simulink model "Kalman_Project"  (R2023a)
settings: Solver=ode45  StartTime=0  StopTime=25  FixedStep=0.002  RelTol=1e-3  AbsTol=1e-6
undefined symbols (not defined in the file or in its folder): J, Reff
libraries: Solver_SF x1, cstblocks x1
settings Model: PacingRate=10  ExtModeTrigMode=oneshot  Creator=ywata  LastModifiedBy=cheho
settings SolverCC: AutoScaleAbsTol=off  AlgebraicLoopSolver=TrustRegion
settings DataIOCC: SaveFormat=Array  SignalLoggingSaveFormat=ModelDataLogs  ReturnWorkspaceOutputs=off  SignalLoggingName=sigsOut
settings OptimizationCC: BlockReduction=off  BooleanDataType=off  ExpressionDepthLimit=2147483647  LifeSpan=inf
settings DebuggingCC: SaveWithParameterizedLinksMsg=none  UnderspecifiedInitializationDetection=Classic  MergeDetectMultiDrivingBlocksExec=none  SignalResolutionControl=TryResolveAllWithWarning  MultiTaskDSMMsg=warning  MultiTaskCondExecSysMsg=none  FcnCallInpInsideContextMsg=warning  UnconnectedInputMsg=warning  UnconnectedOutputMsg=warning  UnconnectedLineMsg=warning  StateNameClashWarn=warning  SFUnexpectedBacktrackingDiag=warning  SFNoUnconditionalDefaultTransitionDiag=warning  SFExecutionAtInitializationDiag=none  ArithmeticOperatorsInVariantConditions=warning
settings HardwareCC: ProdBitPerPointer=32  ProdBitPerSizeT=32  ProdBitPerPtrDiffT=32  ProdLargestAtomicFloat=None  ProdIntDivRoundTo=Undefined  ProdEndianess=Unspecified  ProdWordSize=32  ProdHWDeviceType=32-bit Generic  TargetUnknown=on
settings ModelReferenceCC: PropagateSignalLabelsOutOfModel=off
settings SFSimCC: SimUseLocalCustomCode=off  CustomCodeUndefinedFunction=UseInterfaceOnly
settings RTWCC: TemplateMakefile=grt_vc.tmf  RTWUseLocalCustomCode=off
settings CodeAppCC: StateflowObjectComments=on
settings GRTTargetCC: TargetFcnLib=ansi_tfl_tmw.mat  TargetLangStandard=C89/C90 (ANSI)  CombineOutputUpdateFcns=off  GRTInterface=on
settings ConfigComp: CovMetricSettings=dw  CovSaveCumulativeToWorkspaceVar=on  CovSaveSingleToWorkspaceVar=on  CovExternalEMLEnable=off

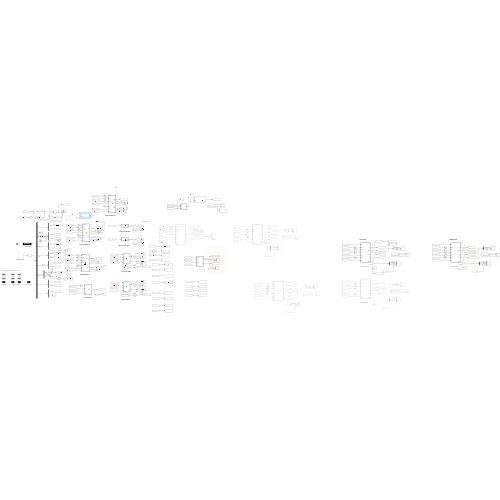
[thumbnail: Simulink's stored preview of the top-level diagram]
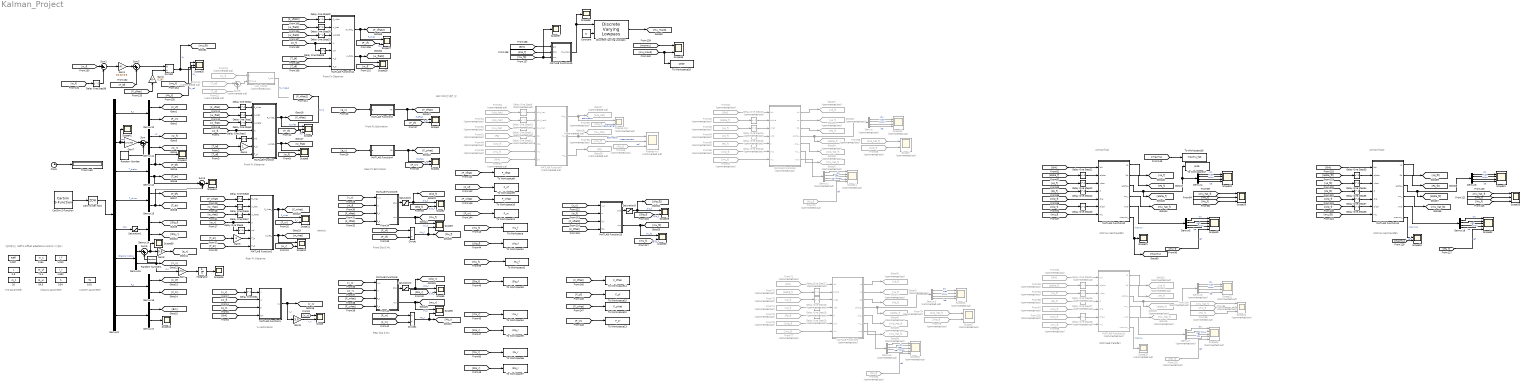
== system Kalman_Project ==
  note: Almost final
  note: IMM(no road transfer)
  note: !실차에서는 Reff와 Offset adaptation control이 필요.!
  note: EKF IMM만 짜면 됨.
  note: Vx estimation
  note: velocity
  note: chassis parameter
  note: tire parameter
  note: system parameter
  note: Front Fx Observer
  note: Rear Fx Observer
  note: Front Fz Estimation
  note: Rear Fz Estimation
  note: Front Slip & Mu
  note: Rear Slip & Mu
  note: IMM(road transfer)
  note: Front Fx Observer
  note: Almost final2
  note: IMM(no road transfer)
  0.01 : DataStoreMemory  DataStoreName=Ts  WriteAfterWriteMsg=warning  InitialValue=0.01  ShowAdditionalParam=off  OutDataTypeStr=double
  0.287 : DataStoreMemory  DataStoreName=Reff  WriteAfterWriteMsg=warning  InitialValue=0.287  ShowAdditionalParam=off  OutDataTypeStr=double
  0.54 : DataStoreMemory  DataStoreName=h  WriteAfterWriteMsg=warning  InitialValue=0.54  ShowAdditionalParam=off  OutDataTypeStr=double
  0.8 : DataStoreMemory  DataStoreName=J  WriteAfterWriteMsg=warning  InitialValue=0.8  ShowAdditionalParam=off  OutDataTypeStr=double
  1.040 : DataStoreMemory  DataStoreName=l_f  WriteAfterWriteMsg=warning  InitialValue=1.040  ShowAdditionalParam=off  OutDataTypeStr=double
  1.560 : DataStoreMemory  DataStoreName=l_r  WriteAfterWriteMsg=warning  InitialValue=1.560  ShowAdditionalParam=off  OutDataTypeStr=double
  1134 : DataStoreMemory  DataStoreName=m_s  WriteAfterWriteMsg=warning  InitialValue=1134  ShowAdditionalParam=off  OutDataTypeStr=double
  16 : DataStoreMemory  DataStoreName=m_t  WriteAfterWriteMsg=warning  InitialValue=16  ShowAdditionalParam=off  OutDataTypeStr=double
  54.5 : DataStoreMemory  DataStoreName=m_ur  WriteAfterWriteMsg=warning  InitialValue=54.5  ShowAdditionalParam=off  OutDataTypeStr=double
  71.4 : DataStoreMemory  DataStoreName=m_uf  WriteAfterWriteMsg=warning  InitialValue=71.4  ShowAdditionalParam=off  OutDataTypeStr=double
  CarSim S-Function : Solver_SF/CarSim S-Function  Priority=1  SIMFILE=simfile.sim  Run_RTs=off  vs_state_ind=Run  StopMode_ind=Vehicle Model
  Clock : Clock
  Constant : Constant  Value=5
  Delay One Step{,1..2,4..6,8,29..30,32,38} (11 alike) : Delay  DelayLength=1
  Delay One Step10 : Delay  Commented=on
  Delay One Step11 : Delay  Commented=on  DelayLength=1
  Delay One Step12 : Delay  Commented=on  DelayLength=1  InitialCondition=[0 0;0 0]
  Delay One Step13 : Delay  Commented=on  DelayLength=1  InitialCondition=[0.25 0.25 0.25 0.25]'
  Delay One Step{14..15,18..19} (4 alike) : Delay  Commented=on  DelayLength=1  InitialCondition=[0 0 0 0;0 0 0 0]
  Delay One Step16 : Delay  Commented=on  DelayLength=1  InitialCondition=[0 0 0 0 0 0 0 0;0 0 0 0 0 0 0 0]
  Delay One Step17 : Delay  Commented=on  DelayLength=1  InitialCondition=[0.25 0.25 0.25 0.25]'
  Delay One Step20 : Delay  Commented=on  DelayLength=1  InitialCondition=[0 0 0 0 0 0 0 0;0 0 0 0 0 0 0 0]
  Delay One Step21 : Delay  DelayLength=1  InitialCondition=[0.25 0.25 0.25 0.25]'
  Delay One Step{22,24..25,34..35,37} (6 alike) : Delay  DelayLength=1  InitialCondition=0
  Delay One Step23 : Delay  Commented=on  DelayLength=1  InitialCondition=[0.25 0.25 0.25 0.25]'
  Delay One Step26 : Delay  Commented=on  DelayLength=1  InitialCondition=0
  Delay One Step27 : Delay  Commented=on  DelayLength=1  InitialCondition=0
  Delay One Step28 : Delay  Commented=on  DelayLength=1  InitialCondition=0
  Delay One Step3 : Delay
  Delay One Step31 : Delay
  Delay One Step33 : Delay  DelayLength=1  InitialCondition=[0.25 0.25 0.25 0.25]'
  Delay One Step36 : Delay  InitialCondition=0
  Delay One Step7 : Delay
  Delay One Step9 : Delay  Commented=on  DelayLength=1
  Demux{,1..3,6..7} (6 alike) : Demux  Commented=on
  Demux{10..17} (8 alike) : Demux  Outputs=[1 1]
      settings: DisplayOption=none
  Demux{4..5,8,18} (4 alike) : Demux
  Demux9 : Demux  Outputs=[2 2 2 2 2 2 2 2]
      settings: DisplayOption=none
  Discrete Varying Lowpass : cstblocks/Linear Parameter Varying/Discrete Varying Lowpass  N=1  w0=0  Ts=0.01
  Divide : Product  Inputs=*/
  Divide1 : Product  Inputs=*/
  Divide2 : Product  Inputs=*/
  From100 : From  Commented=on  GotoTag=mu_hat_f
  From{58,70,80,99,101} (5 alike) : From  Commented=on  GotoTag=Mu_f
  From{49,55,66,68,76,78,97,102} (8 alike) : From  Commented=on  GotoTag=slip_f
  From13 : From  Commented=on  GotoTag=w_f
  From14 : From  Commented=on  GotoTag=T_bf
  From15 : From  Commented=on  GotoTag=T_df
  From{50,56,67,77,95,98} (6 alike) : From  Commented=on  GotoTag=mu_f
  From51 : From  Commented=on  GotoTag=Pp
  From52 : From  Commented=on  GotoTag=mu_hat
  From53 : From  Commented=on  GotoTag=slip_hat
  From54 : From  Commented=on  GotoTag=slip_hat
  From{57,61,71,92} (4 alike) : From  Commented=on  GotoTag=Brk
  From62 : From  Commented=on  GotoTag=alpha_f
  From63 : From  Commented=on  GotoTag=xp_f
  From64 : From  Commented=on  GotoTag=xd_f
  From65 : From  Commented=on  GotoTag=Pp_f
  From69 : From  Commented=on  GotoTag=slip_hat_f
  From72 : From  Commented=on  GotoTag=alpha_f
  From73 : From  Commented=on  GotoTag=xp_f
  From74 : From  Commented=on  GotoTag=xd_f
  From75 : From  Commented=on  GotoTag=Pp_f
  From79 : From  Commented=on  GotoTag=slip_hat_f
  From93 : From  Commented=on  GotoTag=alpha_f
  From94 : From  Commented=on  GotoTag=xp_f
  From96 : From  Commented=on  GotoTag=Pp_f
  Gain : Gain  Gain=1/3.6
  Gain1 : Gain  Gain=1/0.01*0.8
  Gain2 : Gain  Gain=0.287
  Gain3 : Gain
  Gain4 : Gain
  Gain7 : Gain  Gain=2*pi/60
  Gain8 : Gain  Gain=9.8
  Gain9 : Gain  Gain=3.6
  Goto27 : Goto  Commented=on  GotoTag=slip_hat
  Goto28 : Goto  Commented=on  GotoTag=mu_hat
  Goto29 : Goto  Commented=on  GotoTag=Pp
  Goto32 : Goto  Commented=on  GotoTag=mu_hat_f
  Goto33 : Goto  Commented=on  GotoTag=slip_hat_f
  Goto34 : Goto  Commented=on  GotoTag=alpha_f
  Goto35 : Goto  Commented=on  GotoTag=Pp_f
  Goto36 : Goto  Commented=on  GotoTag=xp_f
  Goto37 : Goto  Commented=on  GotoTag=xd_f
  Goto38 : Goto  Commented=on  GotoTag=mu_hat_f
  Goto39 : Goto  Commented=on  GotoTag=slip_hat_f
  Goto40 : Goto  Commented=on  GotoTag=alpha_f
  Goto41 : Goto  Commented=on  GotoTag=Pp_f
  Goto42 : Goto  Commented=on  GotoTag=xp_f
  Goto43 : Goto  Commented=on  GotoTag=xd_f
  Goto45 : Goto  Commented=on  GotoTag=mu_hat_f
  Goto49 : Goto  Commented=on  GotoTag=alpha_f
  Goto50 : Goto  Commented=on  GotoTag=Pp_f
  Goto51 : Goto  Commented=on  GotoTag=xp_f
  Integrator : Integrator
  MATLAB Function : MATLAB Function  TreatAsAtomicUnit=on
  MATLAB Function1 : MATLAB Function  TreatAsAtomicUnit=on
  MATLAB Function10 : MATLAB Function  TreatAsAtomicUnit=on
  MATLAB Function11 : MATLAB Function  Commented=on  TreatAsAtomicUnit=on
  MATLAB Function12 : MATLAB Function  TreatAsAtomicUnit=on
  MATLAB Function13 : MATLAB Function  TreatAsAtomicUnit=on
  MATLAB Function14 : MATLAB Function  TreatAsAtomicUnit=on
  MATLAB Function15 : MATLAB Function  TreatAsAtomicUnit=on
  MATLAB Function2 : MATLAB Function  TreatAsAtomicUnit=on
  MATLAB Function3 : MATLAB Function  TreatAsAtomicUnit=on
  MATLAB Function4 : MATLAB Function  TreatAsAtomicUnit=on
  MATLAB Function5 : MATLAB Function  TreatAsAtomicUnit=on
  MATLAB Function6 : MATLAB Function  TreatAsAtomicUnit=on
  MATLAB Function7 : MATLAB Function  Commented=on  TreatAsAtomicUnit=on
  MATLAB Function8 : MATLAB Function  Commented=on  TreatAsAtomicUnit=on
  MATLAB Function9 : MATLAB Function  Commented=on  TreatAsAtomicUnit=on
  Random Number : RandomNumber  Variance=0.01^2  SampleTime=0.01
  Random Number1 : RandomNumber  Variance=2.25e-8  SampleTime=0.01
  Saturation{,1..3} (4 alike) : Saturate  UpperLimit=1  LowerLimit=-1
  Scope{,1..6,9,11..12,28..30,34,36} (15 alike) : Scope  NumInputPorts=2
  Scope{10,21,26,37..42} (9 alike) : Scope
  Scope13 : Scope  Commented=on  NumInputPorts=4
  Scope14 : Scope  Commented=on  NumInputPorts=5
  Scope15 : Scope  Commented=on  NumInputPorts=4
  Scope16 : Scope  Commented=on  NumInputPorts=5
  Scope17 : Scope  Commented=on  NumInputPorts=2
  Scope18 : Scope  NumInputPorts=4
  Scope19 : Scope  NumInputPorts=5
  Scope{8,20,27,33,35} (5 alike) : Scope  NumInputPorts=3
  Scope22 : Scope  Commented=on  NumInputPorts=4
  Scope23 : Scope  Commented=on  NumInputPorts=5
  Scope24 : Scope  Commented=on  NumInputPorts=3
  Scope25 : Scope  Commented=on
  Scope31 : Scope  NumInputPorts=4
  Scope32 : Scope  NumInputPorts=5
  Scope7 : Scope  Commented=on  NumInputPorts=2
  Sum{,2..3,5} (4 alike) : Sum  Inputs=|++
  Sum1 : Sum  Inputs=|+-
  Sum8 : Sum  Commented=on  Inputs=|++
  Time (sec) : Display
      settings: Format=bank  Decimation=100
  To Workspace : ToWorkspace  VariableName=mu_f  SaveFormat=Timeseries  SampleTime=-1
  To Workspace1 : ToWorkspace  VariableName=slip_f  SaveFormat=Timeseries  SampleTime=-1
  To Workspace10 : ToWorkspace  VariableName=F_xrhat  SaveFormat=Timeseries  SampleTime=-1
  To Workspace11 : ToWorkspace  VariableName=F_xr  SaveFormat=Timeseries  SampleTime=-1
  To Workspace12 : ToWorkspace  VariableName=F_zrhat  SaveFormat=Timeseries  SampleTime=-1
  To Workspace13 : ToWorkspace  VariableName=F_zr  SaveFormat=Timeseries  SampleTime=-1
  To Workspace14 : ToWorkspace  VariableName=F_zfhat  SaveFormat=Timeseries  SampleTime=-1
  To Workspace15 : ToWorkspace  VariableName=F_zf  SaveFormat=Timeseries  SampleTime=-1
  To Workspace16 : ToWorkspace  VariableName=maxmu_hat  SaveFormat=Timeseries  SampleTime=-1
  To Workspace17 : ToWorkspace  VariableName=prob  SaveFormat=Timeseries  SampleTime=-1
  To Workspace18 : ToWorkspace  VariableName=other  SaveFormat=Timeseries  SampleTime=-1
  To Workspace2 : ToWorkspace  VariableName=Mu_f  SaveFormat=Timeseries  SampleTime=-1
  To Workspace3 : ToWorkspace  VariableName=Slip_f  SaveFormat=Timeseries  SampleTime=-1
  To Workspace4 : ToWorkspace  VariableName=mu_r  SaveFormat=Timeseries  SampleTime=-1
  To Workspace5 : ToWorkspace  VariableName=slip_r  SaveFormat=Timeseries  SampleTime=-1
  To Workspace6 : ToWorkspace  VariableName=Mu_r  SaveFormat=Timeseries  SampleTime=-1
  To Workspace7 : ToWorkspace  VariableName=Slip_r  SaveFormat=Timeseries  SampleTime=-1
  To Workspace8 : ToWorkspace  VariableName=F_xfhat  SaveFormat=Timeseries  SampleTime=-1
  To Workspace9 : ToWorkspace  VariableName=F_xf  SaveFormat=Timeseries  SampleTime=-1
  UIO_front2 : Subsystem  Commented=on
  Zero-Order Hold : ZeroOrderHold  SampleTime=0.01
  filtered mu : Scope  Commented=on  NumInputPorts=3
  filtered slip : Scope  Commented=on  NumInputPorts=2
  wires:
  Clock/1 -> Time (sec)/1
  CarSim S-Function/1 -> Zero-Order Hold/1
  Zero-Order Hold/1 -> Demux9/1
  Demux9/1 -> Demux10/1  "F_x"
  Demux10/1 -> [F_xf]
  Demux10/2 -> [F_xr]
  Demux11/2 -> [w_r]
  Demux11/1 -> [w_f]  "wk"
  Demux9/2 -> Scope42/1, Gain7/1  "rpm"
  Gain7/1 -> Sum/1
  Demux12/1 -> Scope40/1, [T_bf]
  Demux12/2 -> Sum3/1, [T_br]
  Demux9/3 -> Demux12/1  "T_brake"
  Demux13/2 -> Sum3/2, [T_dr]
  Demux13/1 -> [T_df]
  Demux9/4 -> Demux13/1  "T_drive"
  Demux14/2 -> [Slip_r]
  Demux14/1 -> [Slip_f]
  Demux9/5 -> Saturation1/1  "slip"
  Demux15/2 -> Gain/1, [V_x]  "V_x"
  Demux15/1 -> Sum5/1
  Demux9/6 -> Demux15/1  "Chassis motion"
  Demux16/2 -> [F_zr]
  Demux16/1 -> [F_zf]
  Demux9/7 -> Demux16/1  "F_z"
  Sum5/1 -> Scope39/1, Gain8/1
  Gain8/1 -> [a_x]
  [w_f] -> MATLAB Function1/2(w)
  [a_x] -> MATLAB Function1/3(a)
  [Brk] -> MATLAB Function1/4(brk)
  Demux9/8 -> Demux17/1
  MATLAB Function1/1(Vx) -> Gain9/1, [v_x]  "v_x"
  [v_x] -> Delay One Step/1
  Delay One Step/1 -> MATLAB Function1/1(v)
  Gain9/1 -> Scope/2  "v_x"
  [V_x] -> Scope/1
  Delay One Step1/1 -> MATLAB Function/5(wd)
  [w_f] -> MATLAB Function/4(w), Delay One Step1/1
  MATLAB Function/2(w_hat_) -> Scope9/1, [w_fhat]
  Delay One Step3/1 -> MATLAB Function/3(w_hatd)
  MATLAB Function/1(F_xhat_) -> Scope8/1, [F_xfhat]  "F_xhat"
  [F_xfhat] -> Delay One Step4/1
  [F_xf] -> Scope8/3  "F_x"
  [w_fhat] -> Delay One Step2/1
  Delay One Step2/1 -> MATLAB Function/2(w_hat)
  Delay One Step4/1 -> MATLAB Function/1(F_xhat)
  Demux17/1 -> [Brk]
  Demux17/2 -> Scope10/1
  [w_f] -> Scope9/2
  [T_bf] -> Gain4/1
  [T_df] -> MATLAB Function/7(T_d)
  From13/1 -> UIO_front2/1(w)
  From14/1 -> Sum8/1
  From15/1 -> Sum8/2
  Sum8/1 -> UIO_front2/2(Torque)
  UIO_front2/1(F_hat) -> ?  "F_x hat_2"
  [w_fhat] -> Delay One Step3/1
  Delay One Step8/1 -> MATLAB Function2/1(F_xhat)
  MATLAB Function2/1(F_xhat_) -> Scope11/1, [F_xrhat]  "F_xhat"
  [F_xr] -> Scope11/2  "F_x"
  [w_rhat] -> Delay One Step6/1
  Delay One Step7/1 -> MATLAB Function2/3(w_hatd)
  [w_rhat] -> Delay One Step7/1
  [F_xrhat] -> Delay One Step8/1
  [w_r] -> Scope12/2
  [T_dr] -> MATLAB Function2/7(T_d)
  [w_r] -> MATLAB Function2/4(w), Delay One Step5/1
  MATLAB Function2/2(w_hat_) -> Scope12/1, [w_rhat]
  Delay One Step6/1 -> MATLAB Function2/2(w_hat)
  [T_br] -> Gain3/1
  Delay One Step5/1 -> MATLAB Function2/5(wd)
  [a_x] -> MATLAB Function3/1(a)
  MATLAB Function3/1(Fz) -> Scope1/1, [F_zfhat]  "F_zfhat"
  MATLAB Function4/1(Fz) -> Scope4/1, [F_zrhat]  "F_zrhat"
  [a_x] -> MATLAB Function4/1(a)
  [F_zf] -> Scope1/2  "F_zf"
  [F_zr] -> Scope4/2  "F_zr"
  [v_x] -> MATLAB Function5/1(v_x)
  [w_f] -> MATLAB Function5/2(w)
  [F_xfhat] -> MATLAB Function5/3(F_x)
  [F_zfhat] -> MATLAB Function5/4(F_z)
  MATLAB Function5/2(mu) -> Scope3/1, [mu_f]  "mu_f"
  [Slip_f] -> Scope2/2  "Silp_f"
  MATLAB Function5/1(slip) -> Saturation/1
  Saturation/1 -> [slip_f], Scope2/1  "slip_f"
  Saturation1/1 -> Demux14/1
  [F_xf] -> Divide/1
  Divide/1 -> Scope3/2, [Mu_f]  "Mu_f"
  [F_zr] -> Divide1/2
  [w_r] -> MATLAB Function6/2(w)
  MATLAB Function6/1(slip) -> Saturation2/1
  [F_xrhat] -> MATLAB Function6/3(F_x)
  [F_zrhat] -> MATLAB Function6/4(F_z)
  [F_xr] -> Divide1/1
  [F_zf] -> Divide/2
  [Slip_r] -> Scope5/2  "Silp_r"
  [v_x] -> MATLAB Function6/1(v_x)
  Saturation2/1 -> [slip_r], Scope5/1  "slip_r"
  MATLAB Function6/2(mu) -> Scope6/1, [mu_r]  "mu_r"
  [mu_f] -> To Workspace/1
  [slip_f] -> To Workspace1/1
  [Slip_f] -> To Workspace3/1
  [slip_r] -> To Workspace5/1
  [Slip_r] -> To Workspace7/1
  [mu_r] -> To Workspace4/1
  Sum/1 -> Demux11/1
  Random Number1/1 -> Sum5/2
  Random Number/1 -> Sum/2
  From49/1 -> MATLAB Function7/5(slip)
  From50/1 -> MATLAB Function7/6(mu)
  MATLAB Function7/1(slip_) -> Goto27/1, filtered slip/1  "estimation"
  MATLAB Function7/2(mu_) -> Goto28/1, filtered mu/1  "estimation"
  MATLAB Function7/3(Pp_) -> Goto29/1
  From52/1 -> Delay One Step11/1
  From53/1 -> Delay One Step9/1
  Delay One Step9/1 -> MATLAB Function7/1(slip_hat)
  From54/1 -> Delay One Step10/1
  Delay One Step10/1 -> MATLAB Function7/2(slip_hatd)
  Delay One Step11/1 -> MATLAB Function7/3(mu_hat)
  From51/1 -> Delay One Step12/1
  Delay One Step12/1 -> MATLAB Function7/4(Pp)
  From55/1 -> filtered slip/2  "measurement"
  From56/1 -> filtered mu/2  "measurement"
  From57/1 -> MATLAB Function7/7(brk)
  [Mu_f] -> To Workspace2/1
  Divide1/1 -> Scope6/2, [Mu_r]  "Mu_r"
  From58/1 -> filtered mu/3  "ref"
  MATLAB Function8/6(mu_) -> Goto32/1
  MATLAB Function8/1(xd) -> Goto37/1
  MATLAB Function8/2(xp) -> Goto36/1
  MATLAB Function8/3(Pp) -> Goto35/1
  MATLAB Function8/4(alpha_) -> Goto34/1, Demux/1
  MATLAB Function8/5(slip_) -> Goto33/1
  From61/1 -> MATLAB Function8/1(brk)
  From62/1 -> Delay One Step13/1
  From63/1 -> Delay One Step14/1
  Delay One Step13/1 -> MATLAB Function8/2(alpha)
  Delay One Step14/1 -> MATLAB Function8/3(xhat)
  From64/1 -> Delay One Step15/1
  Delay One Step15/1 -> MATLAB Function8/4(xdd)
  From65/1 -> Delay One Step16/1
  Delay One Step16/1 -> MATLAB Function8/5(P)
  From66/1 -> MATLAB Function8/6(slip)
  From67/1 -> MATLAB Function8/7(mu)
  From68/1 -> Scope7/2
  From69/1 -> Scope7/1
  Demux/1 -> Scope13/1  "dry"
  Demux/2 -> Scope13/2  "wet"
  Demux/3 -> Scope13/3  "snow"
  Demux/4 -> Scope13/4  "ice"
  MATLAB Function8/7(xmd) -> Demux1/1
  Demux1/1 -> Scope14/1  "dry"
  Demux1/3 -> Scope14/3  "snow"
  Demux1/2 -> Scope14/2  "wet"
  Demux1/4 -> Scope14/4  "ice"
  From70/1 -> Scope14/5  "ref"
  Demux3/1 -> Scope16/1  "dry"
  Demux3/3 -> Scope16/3  "snow"
  Demux3/2 -> Scope16/2  "wet"
  From80/1 -> Scope16/5  "ref"
  MATLAB Function9/7(xmd) -> Demux3/1
  Delay One Step19/1 -> MATLAB Function9/4(xdd)
  MATLAB Function9/1(xd) -> Goto43/1
  MATLAB Function9/4(alpha_) -> Goto40/1, Demux2/1
  MATLAB Function9/5(slip_) -> Goto39/1
  From72/1 -> Delay One Step17/1
  From74/1 -> Delay One Step19/1
  MATLAB Function9/6(mu_) -> Goto38/1
  From71/1 -> MATLAB Function9/1(brk)
  Demux2/1 -> Scope15/1  "dry"
  Delay One Step17/1 -> MATLAB Function9/2(alpha)
  From76/1 -> MATLAB Function9/6(slip)
  From78/1 -> Scope17/2
  Delay One Step18/1 -> MATLAB Function9/3(xhat)
  From79/1 -> Scope17/1
  From75/1 -> Delay One Step20/1
  Demux3/4 -> Scope16/4  "ice"
  From73/1 -> Delay One Step18/1
  MATLAB Function9/3(Pp) -> Goto41/1
  MATLAB Function9/2(xp) -> Goto42/1
  Delay One Step20/1 -> MATLAB Function9/5(P)
  Demux2/3 -> Scope15/3  "snow"
  Demux2/2 -> Scope15/2  "wet"
  Demux2/4 -> Scope15/4  "ice"
  From77/1 -> MATLAB Function9/7(mu)
  Demux5/1 -> Scope19/1  "dry"
  Demux5/3 -> Scope19/3  "snow"
  Demux5/2 -> Scope19/2  "wet"
  [mu_f] -> Scope19/5  "ref"
  MATLAB Function10/5(xmd) -> Demux5/1
  MATLAB Function10/3(alpha_) -> [alpha_f], To Workspace17/1, Demux4/1
  [alpha_f] -> Delay One Step21/1
  MATLAB Function10/4(mu_) -> [mu_hat_f]
  [Brk] -> MATLAB Function10/1(brk)
  Demux4/1 -> Scope18/1  "dry"
  Delay One Step21/1 -> MATLAB Function10/2(alpha)
  [slip_f] -> MATLAB Function10/5(slip)
  [Mu_f] -> Scope20/3
  Delay One Step22/1 -> MATLAB Function10/3(xhat)
  [mu_hat_f] -> Scope20/1
  [Pp_f] -> Delay One Step24/1
  Demux5/4 -> Scope19/4  "ice"
  [xp_f] -> Delay One Step22/1
  MATLAB Function10/2(Pp) -> [Pp_f]
  MATLAB Function10/1(xp) -> [xp_f]
  Delay One Step24/1 -> MATLAB Function10/4(P)
  Demux4/3 -> Scope18/3  "snow"
  Demux4/2 -> Scope18/2  "wet"
  Demux4/4 -> Scope18/4  "ice"
  [mu_f] -> MATLAB Function10/7(mu)
  [slip_f] -> Delay One Step25/1
  Delay One Step25/1 -> MATLAB Function10/6(slipd)
  [mu_f] -> Scope20/2
  MATLAB Function10/6(maxmu_) -> [maxmu], Scope21/1  "maxmu"
  MATLAB Function11/6(maxmu_) -> Scope25/1  "maxmu"
  From98/1 -> MATLAB Function11/7(mu)
  Demux6/4 -> Scope22/4  "ice"
  Delay One Step27/1 -> MATLAB Function11/4(P)
  MATLAB Function11/2(Pp) -> Goto50/1
  Demux6/3 -> Scope22/3  "snow"
  Demux6/1 -> Scope22/1  "dry"
  Delay One Step23/1 -> MATLAB Function11/2(alpha)
  Demux7/4 -> Scope23/4  "ice"
  From100/1 -> Scope24/1
  From96/1 -> Delay One Step27/1
  From99/1 -> Scope24/3
  From94/1 -> Delay One Step26/1
  MATLAB Function11/3(alpha_) -> Goto49/1, Demux6/1
  Delay One Step26/1 -> MATLAB Function11/3(xhat)
  MATLAB Function11/4(mu_) -> Goto45/1
  MATLAB Function11/5(xmd) -> Demux7/1
  From92/1 -> MATLAB Function11/1(brk)
  From97/1 -> MATLAB Function11/5(slip)
  Demux7/3 -> Scope23/3  "snow"
  Demux6/2 -> Scope22/2  "wet"
  Demux7/2 -> Scope23/2  "wet"
  Demux7/1 -> Scope23/1  "dry"
  MATLAB Function11/1(xp) -> Goto51/1
  From101/1 -> Scope23/5  "ref"
  Delay One Step28/1 -> MATLAB Function11/6(slipd)
  From102/1 -> Delay One Step28/1
  From93/1 -> Delay One Step23/1
  From95/1 -> Scope24/2
  Gain/1 -> Integrator/1
  Integrator/1 -> Scope26/1
  [w_fhat2] -> Delay One Step31/1
  [w_f] -> Scope28/2
  [T_bf] -> MATLAB Function12/6(T_b)
  [T_df] -> MATLAB Function12/7(T_d)
  ? -> Scope27/2  "F_x hat_2"
  Delay One Step30/1 -> MATLAB Function12/2(w_hat)
  [w_fhat2] -> Delay One Step30/1
  MATLAB Function12/1(F_xhat_) -> Scope27/1, [F_xfhat2]  "F_xhat"
  Delay One Step31/1 -> MATLAB Function12/3(w_hatd)
  [w_f] -> MATLAB Function12/4(w), Delay One Step29/1
  Delay One Step29/1 -> MATLAB Function12/5(wd)
  [F_xf] -> Scope27/3  "F_x"
  MATLAB Function12/2(w_hat_) -> Scope28/1, [w_fhat2]
  [F_xfhat2] -> Scope8/2  "F_x2"
  [F_xfhat2] -> Delay One Step32/1
  Delay One Step32/1 -> MATLAB Function12/1(F_xhat)
  [F_xfhat2] -> MATLAB Function13/3(F_x)
  [Slip_f] -> Scope29/2  "Silp_f"
  Saturation3/1 -> [slip_f2], Scope29/1  "slip_f"
  [v_x] -> MATLAB Function13/1(v_x)
  MATLAB Function13/2(mu) -> Scope30/1, [mu_f2]  "mu_f2"
  MATLAB Function13/1(slip) -> Saturation3/1
  [w_f] -> MATLAB Function13/2(w)
  [F_zfhat] -> MATLAB Function13/4(F_z)
  [mu_f] -> Scope30/2  "Silp_f"
  Delay One Step36/1 -> MATLAB Function14/6(slipd)
  [mu_f3] -> MATLAB Function14/7(mu)
  Demux8/4 -> Scope31/4  "ice"
  MATLAB Function14/5(xmd) -> Demux18/1
  [slip_f] -> Delay One Step36/1
  [alpha_f2] -> Delay One Step33/1
  Demux8/3 -> Scope31/3  "snow"
  [Pp_f2] -> Delay One Step35/1
  Demux18/4 -> Scope32/4  "ice"
  MATLAB Function14/6(maxmu_) -> Scope34/1  "maxmu2"
  Demux18/1 -> Scope32/1  "dry"
  MATLAB Function14/3(alpha_) -> [alpha_f2], Demux8/1
  Demux18/2 -> Scope32/2  "wet"
  [xp_f2] -> Delay One Step34/1
  [slip_f] -> Delay One Step37/1
  Demux8/2 -> Scope31/2  "wet"
  Delay One Step33/1 -> MATLAB Function14/2(alpha)
  Demux18/3 -> Scope32/3  "snow"
  Delay One Step34/1 -> MATLAB Function14/3(xhat)
  [Mu_f] -> Scope33/3
  [Brk] -> MATLAB Function14/1(brk)
  MATLAB Function14/1(xp) -> [xp_f2]
  Demux8/1 -> Scope31/1  "dry"
  MATLAB Function14/2(Pp) -> [Pp_f2]
  Delay One Step35/1 -> MATLAB Function14/4(P)
  [mu_f] -> Scope33/2
  [mu_hat_f] -> Scope33/1
  [Mu_f] -> Scope32/5  "ref"
  MATLAB Function14/4(mu_) -> [mu_hat_f2]
  [maxmu] -> Scope34/2  "ref"
  Delay One Step37/1 -> MATLAB Function14/5(slip)
  [w_f] -> Sum1/1
  [w_f] -> Delay One Step38/1
  Delay One Step38/1 -> Sum1/2
  Sum1/1 -> Gain1/1
  Gain1/1 -> Sum2/1
  [T_bf] -> Sum2/2
  Sum2/1 -> Divide2/1
  [F_zfhat] -> Gain2/1
  Gain2/1 -> Divide2/2
  Divide2/1 -> [mu_f3], Scope35/1  "Fx"
  [mu_f] -> Scope35/2  "Fx_"
  [Mu_f] -> Scope35/3  "Fx_ref"
  [slip_f] -> MATLAB Function15/2(slip)
  [mu_f3] -> Scope37/1, MATLAB Function15/3(mu)
  [Brk] -> MATLAB Function15/1(brk)
  MATLAB Function15/1(mu_max) -> Scope38/1, Discrete Varying Lowpass/1
  [maxmu] -> Scope36/1
  Discrete Varying Lowpass/1 -> [mu_max3]
  Constant/1 -> Discrete Varying Lowpass/2
  [F_xfhat] -> To Workspace8/1
  [F_xf] -> To Workspace9/1
  [F_xr] -> To Workspace11/1
  [F_xrhat] -> To Workspace10/1
  [F_zrhat] -> To Workspace12/1
  [F_zr] -> To Workspace13/1
  [F_zf] -> To Workspace15/1
  [F_zfhat] -> To Workspace14/1
  [Mu_r] -> To Workspace6/1
  [maxmu] -> To Workspace16/1
  [mu_max3] -> To Workspace18/1, Scope36/2
  Gain3/1 -> MATLAB Function2/6(T_b)
  Gain4/1 -> MATLAB Function/6(T_b)
  Sum3/1 -> Scope41/1

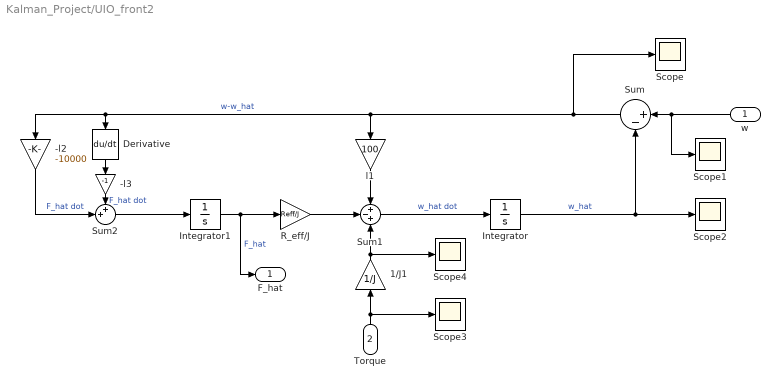
== system Kalman_Project/UIO_front2 ==
  w : Inport
  Torque : Inport  Port=2
  -l2 : Gain  Gain=-10000
  -l3 : Gain  Gain=-1
  1/J1 : Gain  Gain=1/J
  Derivative : Derivative
  Integrator : Integrator
  Integrator1 : Integrator
  R_eff/J : Gain  Gain=Reff/J
  Scope{,1..4} (5 alike) : Scope
  Sum : Sum  Inputs=|+-
  Sum1 : Sum  Inputs=+-+
  Sum2 : Sum  Inputs=++|
  l1 : Gain  Gain=100
  F_hat : Outport
  wires:
  w/1 -> Scope1/1, Sum/1
  Integrator/1 -> Sum/2, Scope2/1  "w_hat"
  Sum1/1 -> Integrator/1  "w_hat dot"
  Sum/1 -> -l2/1, Derivative/1, l1/1, Scope/1  "w-w_hat"
  l1/1 -> Sum1/1
  -l2/1 -> Sum2/2  "F_hat dot"
  Integrator1/1 -> F_hat/1, R_eff/J/1  "F_hat"
  R_eff/J/1 -> Sum1/2
  Torque/1 -> 1/J1/1, Scope3/1
  1/J1/1 -> Sum1/3, Scope4/1
  Sum2/1 -> Integrator1/1
  Derivative/1 -> -l3/1
  -l3/1 -> Sum2/1  "F_hat dot"

== matlab function Kalman_Project/MATLAB Function6 ==
  data: v_x input; w input; slip output; F_x input; F_z input; Reff data_store_memory; mu output
function [slip,mu] = fcn(v_x,w,F_x,F_z)
global Reff;

slip = (w*Reff - v_x)/max(v_x,w*Reff);
mu = F_x/F_z;

end

== matlab function Kalman_Project/MATLAB Function7 ==
  data: slip_hat input; slip_hatd input; slip_ output; mu_hat input; Pp input; slip input; mu input; mu_ output; Pp_ output; brk input
function [slip_, mu_,Pp_] = fcn(slip_hat,slip_hatd,mu_hat,Pp,slip,mu,brk)
% Dry Asphalt EFK
if brk == 0
    slip_ = 0; mu_ = 0; Pp_ = [0 0;0 0];
else
    % Tuning Params.
    Q = [0.5 0; 0 0.01]; R = [0.1 0; 0 10000000];
    
    x = [slip_hat; mu_hat];
    y = [slip; mu];
    F = [1 0; ddf(x(1))*(x(1)-slip_hatd)+df(x(1)) 1];  L = eye(2);
    H = eye(2); M = eye(2);
    
    xm = [x(1); x(2)+df(x(1))*(x(1)-slip_hatd)];
    Pm = F*Pp*F'+L*Q*L';
    K = Pm*H'/(H*Pm*H'+M*R*M');
    xp = xm + K*(y-xm);
    Pp = (eye(2)-K*H)*Pm;
    
    %out
    slip_ = xp(1);
    mu_ = xp(2);
    Pp_ = Pp;
end

end

function dF = df(x)
B = 10; C = 1.9; D = 1; E = 0.97;
% B = 5; C = 2; D = 0.3; E = 1;

dF = (C*D*cos(C*atan(B*x + E*(atan(B*x) - B*x)))*(B - E*(B - B/(B^2*x^2 + 1))))/((B*x + E*(atan(B*x) - B*x))^2 + 1);

end

function ddF = ddf(x)

B = 10; C = 1.9; D = 1; E = 0.97;
% B = 5; C = 2; D = 0.3; E = 1;

ddF = - (C^2*D*sin(C*atan(B*x + E*(atan(B*x) - B*x)))*(B - E*(B - B/(B^2*x^2 + 1)))^2)/((B*x + E*(atan(B*x) - B*x))^2 + 1)^2 ...
- (2*C*D*cos(C*atan(B*x + E*(atan(B*x) - B*x)))*(B*x + E*(atan(B*x) - B*x))*(B - E*(B - B/(B^2*x^2 + 1)))^2)/((B*x + E*(atan(B*x) - B*x))^2 + 1)^2 ...
- (2*B^3*C*D*E*x*cos(C*atan(B*x + E*(atan(B*x) - B*x))))/((B^2*x^2 + 1)^2*((B*x + E*(atan(B*x) - B*x))^2 + 1));

end

== matlab function Kalman_Project/MATLAB Function8 ==
  data: xd output; xp output; Pp output; alpha_ output; slip_ output; brk input; alpha input; xhat input; xdd input; P input; slip input; mu input; mu_ output; xmd output
function [xd,xp,Pp,alpha_,slip_,mu_,xmd] = fcn(brk,alpha,xhat,xdd,P,slip,mu)
% Dry Asphalt EFK
y = [slip; mu];
if brk == 0
    slip_ = 0; mu_ = 0; Pp = P; alpha_ = [0.25 0.25 0.25 0.25]'; xd = xdd; xp = xd; xmd = [0 0 0 0];
else
    % Tuning Params.
    % Pi = [0.9 0.08 0.01 0.01; 0.08 0.9 0.01 0.01; 0.01 0.01 0.9 0.08; 0.01 0.01 0.08 0.9]; M = length(Pi(1,:));
    Pi = eye(4); M = length(Pi(1,:));
    Q = [0.1 0; 0 0.000000001]; R = [0.01 0; 0 0.1];

    % Beta ji table [4x4]
    Beta = zeros(M,M);
    for i = 1:M
        Beta(:,i) = alpha.*Pi(:,i)/sum(alpha.*Pi(:,i));
    end

    % x_hat k-1 ++ [2x4]
    xd = xhat*Beta;

    % P k-1 ++ [2x8]
    Pd = zeros(2,2*M);
    for i = 1:M
        for j = 1:M
            Pd(:,2*i-1:2*i) = Pd(:,2*i-1:2*i) + Beta(j,i)*(P(:,2*j-1:2*j)+(xhat(:,j)-xd(:,j))*(xhat(:,j)-xd(:,j))');
        end
    end

    % EKF
    xmd = zeros(1,M); %
    xp = zeros(2,M);
    Pp = zeros(2,2*M);
    N = zeros(1,M);
    rd = zeros(2,M); %
    Sd = zeros(2,2*M); %
    dF = zeros(1,M); %
    ddF = zeros(1,M); %
    for i = 1:M
        F = [1 0; ddf(xd(1,i),i)*(xd(1,i)-xdd(1,i))+df(xd(1,i),i) 1]; L = eye(2);
        H = eye(2); M_ = eye(2);
        dF(i) = df(xd(1,i),i); ddF(i) = ddf(xd(1,i),i); %
        xm = [xd(1,i); xd(2,i)+df(xd(1,i),i)*(xd(1,i)-xdd(1,i))];
        xmd(i) = xm(2); %
        Pm = F*Pd(:,2*i-1:2*i)*F'+L*Q*L';
        r = y - xm;
        rd(:,i) = r; %
        S = H*Pm*H'+M_*R*M_';
        Sd(:,2*i-1:2*i) = S;
        K = Pm*H'/S;
        xp(:,i) = xm + K*r;
        Pp(:,2*i-1:2*i) = (eye(2)-K*H)*Pm;
        % N(i) = exp(-[0;r(2)]'/S*[0;r(2)]/2)/(2*pi*det(S)^0.5);
        N(i) = exp(-r(2)'/S(2,2)*r(2)/2)/(2*pi*det(S(2,2))^0.5);
    end
    
    % alpha
    alpha_ = zeros(4,1);
    for i = 1:M
        alpha_(i) = N*(alpha.*Pi(:,i));
    end
    alpha_ = alpha_/sum(alpha_);

    % Overall posterior
    slip_ = xp(1,:)*alpha_;
    mu_ = xp(2,:)*alpha_;
end
end

function dF = df(x,i)
B = [10 12 5 4]'; C = [1.9 2.3 2 2]'; D = [1 0.82 0.3 0.1]'; E = [0.97 1 1 1]';
B = B(i); C = C(i); D = D(i); E = E(i);

dF = (C*D*cos(C*atan(B*x + E*(atan(B*x) - B*x)))*(B - E*(B - B/(B^2*x^2 + 1))))/((B*x + E*(atan(B*x) - B*x))^2 + 1);

end

function ddF = ddf(x,i)

B = [10 12 5 4]'; C = [1.9 2.3 2 2]'; D = [1 0.82 0.3 0.1]'; E = [0.97 1 1 1]';
B = B(i); C = C(i); D = D(i); E = E(i);

ddF = - (C^2*D*sin(C*atan(B*x + E*(atan(B*x) - B*x)))*(B - E*(B - B/(B^2*x^2 + 1)))^2)/((B*x + E*(atan(B*x) - B*x))^2 + 1)^2 ...
- (2*C*D*cos(C*atan(B*x + E*(atan(B*x) - B*x)))*(B*x + E*(atan(B*x) - B*x))*(B - E*(B - B/(B^2*x^2 + 1)))^2)/((B*x + E*(atan(B*x) - B*x))^2 + 1)^2 ...
- (2*B^3*C*D*E*x*cos(C*atan(B*x + E*(atan(B*x) - B*x))))/((B^2*x^2 + 1)^2*((B*x + E*(atan(B*x) - B*x))^2 + 1));

end

== matlab function Kalman_Project/MATLAB Function9 ==
  data: xd output; xp output; Pp output; alpha_ output; slip_ output; brk input; alpha input; xhat input; xdd input; P input; slip input; mu input; mu_ output; xmd output
function [xd,xp,Pp,alpha_,slip_,mu_,xmd] = fcn(brk,alpha,xhat,xdd,P,slip,mu)
% Dry Asphalt EFK
y = [slip; mu];
if brk == 0
    slip_ = 0; mu_ = 0; Pp = P; alpha_ = [0.25 0.25 0.25 0.25]'; xd = xdd; xp = xd; xmd = [0 0 0 0];
else
    % Tuning Params.
    % Pi = [0.9 0.08 0.01 0.01; 0.08 0.9 0.01 0.01; 0.01 0.01 0.9 0.08; 0.01 0.01 0.08 0.9]; M = length(Pi(1,:));
    Pi = eye(4); M = length(Pi(1,:));
    Q = [0.05 0; 0 0.01]; R = [0.01 0; 0 1];

    % Beta ji table [4x4]
    Beta = zeros(M,M);
    for i = 1:M
        Beta(:,i) = alpha.*Pi(:,i)/sum(alpha.*Pi(:,i));
    end

    % x_hat k-1 ++ [2x4]
    xd = xhat*Beta;

    % P k-1 ++ [2x8]
    Pd = zeros(2,2*M);
    for i = 1:M
        for j = 1:M
            Pd(:,2*i-1:2*i) = Pd(:,2*i-1:2*i) + Beta(j,i)*(P(:,2*i-1:2*i)+(xhat(:,j)-xd(:,j))*(xhat(:,j)-xd(:,j))');
        end
    end

    % EKF
    xmd = zeros(1,M); %
    xp = zeros(2,M);
    Pp = zeros(2,2*M);
    N = zeros(1,M);
    rd = zeros(2,M); %
    Sd = zeros(2,2*M); %
    % Fd
    for i = 1:M
        F = [1 0; df(xd(1,i),i) 1]; L = eye(2);
        H = eye(2); M_ = eye(2);

        xm = [xd(1,i); f(xd(1,i),i)+df(xd(1,i),i)*(xd(1,i)-xdd(1,i))];
        xmd(i) = xm(2); %
        Pm = F*Pd(:,2*i-1:2*i)*F'+L*Q*L';
        r = y - xm;
        rd(:,i) = r; %
        S = H*Pm*H'+M_*R*M_';
        Sd(:,2*i-1:2*i) = S;
        K = Pm*H'/S;
        xp(:,i) = xm + K*r;
        Pp(:,2*i-1:2*i) = (eye(2)-K*H)*Pm;
        % N(i) = exp(-[0;r(2)]'/S*[0;r(2)]/2)/(2*pi*det(S)^0.5);
        N(i) = exp(-r'/S*r/2)/(2*pi*det(S)^0.5);
    end
    
    % alpha
    alpha_ = zeros(4,1);
    for i = 1:M
        alpha_(i) = N*(alpha.*Pi(:,i));
    end
    alpha_ = alpha_/sum(alpha_);

    % Overall posterior
    slip_ = xp(1,:)*alpha_;
    mu_ = xp(2,:)*alpha_;
end
end

function F = f(x,i)
B = [10 12 5 4]'; C = [1.9 2.3 2 2]'; D = [1 0.82 0.3 0.1]'; E = [0.97 1 1 1]';
B = B(i); C = C(i); D = D(i); E = E(i);

F = D*sin(C*atan(B*x-E*(B*x-atan(B*x))));

end

function dF = df(x,i)
B = [10 12 5 4]'; C = [1.9 2.3 2 2]'; D = [1 0.82 0.3 0.1]'; E = [0.97 1 1 1]';
B = B(i); C = C(i); D = D(i); E = E(i);

dF = (C*D*cos(C*atan(B*x + E*(atan(B*x) - B*x)))*(B - E*(B - B/(B^2*x^2 + 1))))/((B*x + E*(atan(B*x) - B*x))^2 + 1);

end

function ddF = ddf(x,i)

B = [10 12 5 4]'; C = [1.9 2.3 2 2]'; D = [1 0.82 0.3 0.1]'; E = [0.97 1 1 1]';
B = B(i); C = C(i); D = D(i); E = E(i);

ddF = - (C^2*D*sin(C*atan(B*x + E*(atan(B*x) - B*x)))*(B - E*(B - B/(B^2*x^2 + 1)))^2)/((B*x + E*(atan(B*x) - B*x))^2 + 1)^2 ...
- (2*C*D*cos(C*atan(B*x + E*(atan(B*x) - B*x)))*(B*x + E*(atan(B*x) - B*x))*(B - E*(B - B/(B^2*x^2 + 1)))^2)/((B*x + E*(atan(B*x) - B*x))^2 + 1)^2 ...
- (2*B^3*C*D*E*x*cos(C*atan(B*x + E*(atan(B*x) - B*x))))/((B^2*x^2 + 1)^2*((B*x + E*(atan(B*x) - B*x))^2 + 1));

end

== matlab function Kalman_Project/MATLAB Function10 ==
  data: xp output; Pp output; alpha_ output; brk input; alpha input; xhat input; P input; slip input; slipd input; mu input; mu_ output; xmd output; maxmu_ output
function [xp,Pp,alpha_,mu_,xmd,maxmu_] = fcn(brk,alpha,xhat,P,slip,slipd,mu)
% Dry Asphalt EFK
y = mu;
if brk == 0
    mu_ = 0; Pp = [0 0 0 0]; alpha_ = [0.25 0.25 0.25 0.25]'; xp = [0 0 0 0]; xmd = [0 0 0 0]; maxmu_ = 0;
else
    % Tuning Params.
    % Pi = [0.9999 0.00005 0.00003 0.00002; 0.00005 0.9999 0.00003 0.00002; 0.00002 0.00003 0.9999 0.00005; 0.00002 0.00003 0.00005 0.9999]; M = length(Pi(1,:));
    Pi = eye(4); M = length(Pi(1,:));
    Q = 0.000001; R = 1;

    % Beta ji table [4x4]
    
    Beta = zeros(M,M);
    for i = 1:M
        Beta(:,i) = alpha.*Pi(:,i)/sum(alpha.*Pi(:,i));
    end
    alpha = alpha+0.001;
    % x_hat k-1 ++ [1x4]
    xd = xhat*Beta;
    % xd = [0 0 0 0];

    % P k-1 ++ [1x4]
    Pd = zeros(1,M);
    for i = 1:M
        for j = 1:M
            Pd(i) = Pd(i) + Beta(j,i)*(P(j)+(xhat(j)-xd(j))*(xhat(j)-xd(j))');
        end
    end

    % EKF
    xmd = zeros(1,M); %
    xp = zeros(1,M);
    Pp = zeros(1,4);
    N = zeros(1,M);
    rd = zeros(1,M); %
    Sd = zeros(1,M); %
    dF = zeros(1,M); %
    for i = 1:M
        F = 1; H = 1;
        dF(i) = df(xd(i),i); %
        xm = f(slip,i); %
        % xm = xd(i)+df(slip,i)*(slip-slipd);
        xmd(i) = xm; %
        Pm = F*Pd(i)*F'+Q;
        r = y - xm;
        rd(i) = r; %
        S = H*Pm*H'+R;
        Sd(i) = S;
        K = Pm*H'/S;
        xp(i) = xm + K*r;
        Pp(i) = (1-K*H)*Pm;
        % N(i) = exp(-[0;r(2)]'/S*[0;r(2)]/2)/(2*pi*det(S)^0.5);
        N(i) = exp(-r/S*r/2)/((2*pi)^0.5*det(S)^0.5);
    end
    
    % alpha
    alpha_ = zeros(4,1);
    for i = 1:M
        alpha_(i) = N*(alpha.*Pi(:,i));
    end
    alpha_ = alpha_/sum(alpha_);

    % Overall posterior
    mu_ = xp*alpha_;
    D = [1 0.82 0.3 0.1];
    maxmu_ = D*alpha_;
end
end

function F = f(x,i)
B = [10 12 5 4]'; C = [1.9 2.3 2 2]'; D = [1 0.82 0.3 0.1]'; E = [0.97 1 1 1]';
B = B(i); C = C(i); D = D(i); E = E(i);

F = D*sin(C*atan(B*x-E*(B*x-atan(B*x))));

end

function dF = df(x,i)
B = [10 12 5 4]'; C = [1.9 2.3 2 2]'; D = [1 0.82 0.3 0.1]'; E = [0.97 1 1 1]';
B = B(i); C = C(i); D = D(i); E = E(i);

dF = (C*D*cos(C*atan(B*x + E*(atan(B*x) - B*x)))*(B - E*(B - B/(B^2*x^2 + 1))))/((B*x + E*(atan(B*x) - B*x))^2 + 1);

end

function ddF = ddf(x,i)

B = [10 12 5 4]'; C = [1.9 2.3 2 2]'; D = [1 0.82 0.3 0.1]'; E = [0.97 1 1 1]';
B = B(i); C = C(i); D = D(i); E = E(i);

ddF = - (C^2*D*sin(C*atan(B*x + E*(atan(B*x) - B*x)))*(B - E*(B - B/(B^2*x^2 + 1)))^2)/((B*x + E*(atan(B*x) - B*x))^2 + 1)^2 ...
- (2*C*D*cos(C*atan(B*x + E*(atan(B*x) - B*x)))*(B*x + E*(atan(B*x) - B*x))*(B - E*(B - B/(B^2*x^2 + 1)))^2)/((B*x + E*(atan(B*x) - B*x))^2 + 1)^2 ...
- (2*B^3*C*D*E*x*cos(C*atan(B*x + E*(atan(B*x) - B*x))))/((B^2*x^2 + 1)^2*((B*x + E*(atan(B*x) - B*x))^2 + 1));

end

== matlab function Kalman_Project/MATLAB Function11 ==
  data: xp output; Pp output; alpha_ output; brk input; alpha input; xhat input; P input; slip input; slipd input; mu input; mu_ output; xmd output; maxmu_ output
function [xp,Pp,alpha_,mu_,xmd,maxmu_] = fcn(brk,alpha,xhat,P,slip,slipd,mu)
% Dry Asphalt EFK
y = mu;
if brk == 0
    mu_ = 0; Pp = [0 0 0 0]; alpha_ = [0.25 0.25 0.25 0.25]'; xp = [0 0 0 0]; xmd = [0 0 0 0]; maxmu_ = 0;
else
    % Tuning Params.
    % Pi = [0.999 0.0005 0.0003 0.0002; 0.0005 0.999 0.0003 0.0002; 0.0002 0.0003 0.999 0.0005; 0.0002 0.0003 0.0005 0.999]; M = length(Pi(1,:));
    Pi = eye(4); M = length(Pi(1,:));
    Q = 0.0001; R = 1;
    alpha = alpha + 0.002;
    % Beta ji table [4x4]
    Beta = zeros(M,M);
    for i = 1:M
        Beta(:,i) = alpha.*Pi(:,i)/sum(alpha.*Pi(:,i));
    end

    % x_hat k-1 ++ [1x4]
    xd = xhat*Beta;
    % xd = [0 0 0 0];

    % P k-1 ++ [1x4]
    Pd = zeros(1,M);
    for i = 1:M
        for j = 1:M
            Pd(i) = Pd(i) + Beta(j,i)*(P(j)+(xhat(j)-xd(j))*(xhat(j)-xd(j))');
        end
    end

    % EKF
    xmd = zeros(1,M); %
    xp = zeros(1,M);
    Pp = zeros(1,4);
    N = zeros(1,M);
    rd = zeros(1,M); %
    Sd = zeros(1,M); %
    dF = zeros(1,M); %
    for i = 1:M
        F = 1; H = 1;
        dF(i) = df(xd(i),i); %
        xm = xd(i)+df(slip,i)*(slip-slipd);
        xmd(i) = xm; %
        Pm = F*Pd(i)*F'+Q;
        r = y - xm;
        rd(i) = r; %
        S = H*Pm*H'+R;
        Sd(i) = S;
        K = Pm*H'/S;
        xp(i) = xm + K*r;
        Pp(i) = (1-K*H)*Pm;
        % N(i) = exp(-[0;r(2)]'/S*[0;r(2)]/2)/(2*pi*det(S)^0.5);
        N(i) = exp(-r/S*r/2)/((2*pi)^0.5*det(S)^0.5);
    end
    
    % alpha
    alpha_ = zeros(4,1);
    for i = 1:M
        alpha_(i) = N*(alpha.*Pi(:,i));
    end
    alpha_ = alpha_/sum(alpha_);

    % Overall posterior
    mu_ = xp*alpha_;
    D = [1 0.82 0.3 0.1];
    maxmu_ = D*alpha_;
    
end
end

% function F = f(x,i)
% B = [10 12 5 4]'; C = [1.9 2.3 2 2]'; D = [1 0.82 0.3 0.1]'; E = [0.97 1 1 1]';
% B = B(i); C = C(i); D = D(i); E = E(i);
% 
% F = D*sin(C*atan(B*x-E*(B*x-atan(B*x))));
% 
% end

function dF = df(x,i)
B = [10 12 5 4]'; C = [1.9 2.3 2 2]'; D = [1 0.82 0.3 0.1]'; E = [0.97 1 1 1]';
B = B(i); C = C(i); D = D(i); E = E(i);

dF = (C*D*cos(C*atan(B*x + E*(atan(B*x) - B*x)))*(B - E*(B - B/(B^2*x^2 + 1))))/((B*x + E*(atan(B*x) - B*x))^2 + 1);

end

function ddF = ddf(x,i)

B = [10 12 5 4]'; C = [1.9 2.3 2 2]'; D = [1 0.82 0.3 0.1]'; E = [0.97 1 1 1]';
B = B(i); C = C(i); D = D(i); E = E(i);

ddF = - (C^2*D*sin(C*atan(B*x + E*(atan(B*x) - B*x)))*(B - E*(B - B/(B^2*x^2 + 1)))^2)/((B*x + E*(atan(B*x) - B*x))^2 + 1)^2 ...
- (2*C*D*cos(C*atan(B*x + E*(atan(B*x) - B*x)))*(B*x + E*(atan(B*x) - B*x))*(B - E*(B - B/(B^2*x^2 + 1)))^2)/((B*x + E*(atan(B*x) - B*x))^2 + 1)^2 ...
- (2*B^3*C*D*E*x*cos(C*atan(B*x + E*(atan(B*x) - B*x))))/((B^2*x^2 + 1)^2*((B*x + E*(atan(B*x) - B*x))^2 + 1));

end

== matlab function Kalman_Project/MATLAB Function12 ==
  data: F_xhat input; F_xhat_ output; w_hat input; w_hatd input; w_hat_ output; w input; wd input; T_b input; T_d input; Reff data_store_memory; J data_store_memory; Ts data_store_memory
function [F_xhat_,w_hat_]= UIO_f(F_xhat,w_hat,w_hatd,w,wd,T_b,T_d)

global Reff J Ts;
l1 = 100; l2 = 10000; l3 = 0;

w_hatdot = 1/J*(T_b+T_d) - Reff/J*F_xhat + l1*(w-w_hat);
w_hat_ = w_hat + w_hatdot*Ts;

F_xhatdot = -l2*(w-w_hat) - l3*((w-wd)/Ts - (w_hat-w_hatd)/Ts);
F_xhat_ = F_xhat + F_xhatdot*Ts;




end

== matlab function Kalman_Project/MATLAB Function13 ==
  data: v_x input; w input; slip output; F_x input; F_z input; Reff data_store_memory; mu output
function [slip,mu] = fcn(v_x,w,F_x,F_z)
global Reff;

slip = (w*Reff - v_x)/max(v_x,w*Reff);
mu = F_x/F_z;

end

== matlab function Kalman_Project/MATLAB Function14 ==
  data: xp output; Pp output; alpha_ output; brk input; alpha input; xhat input; P input; slip input; slipd input; mu input; mu_ output; xmd output; maxmu_ output
function [xp,Pp,alpha_,mu_,xmd,maxmu_] = fcn(brk,alpha,xhat,P,slip,slipd,mu)
% Dry Asphalt EFK
y = mu;
if brk == 0
    mu_ = 0; Pp = [0 0 0 0]; alpha_ = [0.25 0.25 0.25 0.25]'; xp = [0 0 0 0]; xmd = [0 0 0 0]; maxmu_ = 0;
else
    % Tuning Params.
    % Pi = [0.9999 0.00005 0.00003 0.00002; 0.00005 0.9999 0.00003 0.00002; 0.00002 0.00003 0.9999 0.00005; 0.00002 0.00003 0.00005 0.9999]; M = length(Pi(1,:));
    Pi = eye(4); M = length(Pi(1,:));
    Q = 0.000001; R = 1;

    % Beta ji table [4x4]
    
    Beta = zeros(M,M);
    for i = 1:M
        Beta(:,i) = alpha.*Pi(:,i)/sum(alpha.*Pi(:,i));
    end
    alpha = alpha+0.001;
    % x_hat k-1 ++ [1x4]
    xd = xhat*Beta;
    % xd = [0 0 0 0];

    % P k-1 ++ [1x4]
    Pd = zeros(1,M);
    for i = 1:M
        for j = 1:M
            Pd(i) = Pd(i) + Beta(j,i)*(P(j)+(xhat(j)-xd(j))*(xhat(j)-xd(j))');
        end
    end

    % EKF
    xmd = zeros(1,M); %
    xp = zeros(1,M);
    Pp = zeros(1,4);
    N = zeros(1,M);
    rd = zeros(1,M); %
    Sd = zeros(1,M); %
    dF = zeros(1,M); %
    for i = 1:M
        F = 1; H = 1;
        dF(i) = df(xd(i),i); %
        xm = xd(i)+df(slip,i)*(slip-slipd);
        xmd(i) = xm; %
        Pm = F*Pd(i)*F'+Q;
        r = y - xm;
        rd(i) = r; %
        S = H*Pm*H'+R;
        Sd(i) = S;
        K = Pm*H'/S;
        xp(i) = xm + K*r;
        Pp(i) = (1-K*H)*Pm;
        % N(i) = exp(-[0;r(2)]'/S*[0;r(2)]/2)/(2*pi*det(S)^0.5);
        N(i) = exp(-r/S*r/2)/((2*pi)^0.5*det(S)^0.5);
    end
    
    % alpha
    alpha_ = zeros(4,1);
    for i = 1:M
        alpha_(i) = N*(alpha.*Pi(:,i));
    end
    alpha_ = alpha_/sum(alpha_);

    % Overall posterior
    mu_ = xp*alpha_;
    D = [1 0.82 0.3 0.1];
    maxmu_ = D*alpha_;
end
end

function F = f(x,i)
B = [10 12 5 4]'; C = [1.9 2.3 2 2]'; D = [1 0.82 0.3 0.1]'; E = [0.97 1 1 1]';
B = B(i); C = C(i); D = D(i); E = E(i);

F = D*sin(C*atan(B*x-E*(B*x-atan(B*x))));

end

function dF = df(x,i)
B = [10 12 5 4]'; C = [1.9 2.3 2 2]'; D = [1 0.82 0.3 0.1]'; E = [0.97 1 1 1]';
B = B(i); C = C(i); D = D(i); E = E(i);

dF = (C*D*cos(C*atan(B*x + E*(atan(B*x) - B*x)))*(B - E*(B - B/(B^2*x^2 + 1))))/((B*x + E*(atan(B*x) - B*x))^2 + 1);

end

function ddF = ddf(x,i)

B = [10 12 5 4]'; C = [1.9 2.3 2 2]'; D = [1 0.82 0.3 0.1]'; E = [0.97 1 1 1]';
B = B(i); C = C(i); D = D(i); E = E(i);

ddF = - (C^2*D*sin(C*atan(B*x + E*(atan(B*x) - B*x)))*(B - E*(B - B/(B^2*x^2 + 1)))^2)/((B*x + E*(atan(B*x) - B*x))^2 + 1)^2 ...
- (2*C*D*cos(C*atan(B*x + E*(atan(B*x) - B*x)))*(B*x + E*(atan(B*x) - B*x))*(B - E*(B - B/(B^2*x^2 + 1)))^2)/((B*x + E*(atan(B*x) - B*x))^2 + 1)^2 ...
- (2*B^3*C*D*E*x*cos(C*atan(B*x + E*(atan(B*x) - B*x))))/((B^2*x^2 + 1)^2*((B*x + E*(atan(B*x) - B*x))^2 + 1));

end

== matlab function Kalman_Project/MATLAB Function1 ==
  data: v input; w input; Vx output; a input; brk input; Reff data_store_memory; Ts data_store_memory
function Vx = fcn(v,w,a,brk)
global Ts Reff;

if brk == 0
    Vx = (w*Reff + v)/2;
else
    Vx = v + a*Ts;
end
end

== matlab function Kalman_Project/MATLAB Function15 ==
  data: brk input; slip input; mu_max output; mu input
function mu_max = fcn(brk,slip,mu)
slip = -slip;
mu = -mu;
if brk == 0
    mu_max = 0;
else
    c1 = [1.28 0.857 1.197 0.4 0.195 0.05]; 
    c2 = [23.99 33.82 25.17 33.71 94.13 306.39];
    c3 = [0.52 0.35 0.54 0.12 0.065 0.001];
    
    M_std = zeros(1,6);
    for i = 1:6
        mu_std = c1(i)*(1-exp(-c2(i).*slip))-c3(i).*slip;
        M_std(i) = mu_std*slip;
    end
    M = mu*slip;
    
    M_diff = abs(M_std-M);
    [~,idx] = min(M_diff);
    
    mu_max = c1(idx) - c3(idx)/c2(idx)*(1+log(c1(idx)*c2(idx)/c3(idx)));
end

end

== matlab function Kalman_Project/MATLAB Function ==
  data: F_xhat input; F_xhat_ output; w_hat input; w_hatd input; w_hat_ output; w input; wd input; T_b input; T_d input; Reff data_store_memory; J data_store_memory; Ts data_store_memory
function [F_xhat_,w_hat_]= UIO_f(F_xhat,w_hat,w_hatd,w,wd,T_b,T_d)

global Reff J Ts;
l1 = 1; l2 = 1000; l3 = 100;

w_hatdot = 1/J*(T_b+T_d) - Reff/J*F_xhat + l1*(w-w_hat);
w_hat_ = w_hat + w_hatdot*Ts;

F_xhatdot = -l2*(w-w_hat) - l3*((w-wd)/Ts - (w_hat-w_hatd)/Ts);
F_xhat_ = F_xhat + F_xhatdot*Ts;




end

== matlab function Kalman_Project/MATLAB Function2 ==
  data: F_xhat input; F_xhat_ output; w_hat input; w_hatd input; w_hat_ output; w input; wd input; T_b input; T_d input; Reff data_store_memory; J data_store_memory; Ts data_store_memory
function [F_xhat_,w_hat_]= UIO_r(F_xhat,w_hat,w_hatd,w,wd,T_b,T_d)

global Reff J Ts;
l1 = 1; l2 = 1000; l3 = 100;

w_hatdot = 1/J*(T_b+T_d) - Reff/J*F_xhat + l1*(w-w_hat);
w_hat_ = w_hat + w_hatdot*Ts;

F_xhatdot = -l2*(w-w_hat) - l3*((w-wd)/Ts - (w_hat-w_hatd)/Ts);
F_xhat_ = F_xhat + F_xhatdot*Ts;




end

== matlab function Kalman_Project/MATLAB Function3 ==
  data: Fz output; a input; l_r data_store_memory; h data_store_memory; m_s data_store_memory; m_uf data_store_memory; l_f data_store_memory; m_t data_store_memory
function Fz = fcn(a)
global m_s m_uf l_f l_r h m_t;

Fz = ((m_s*l_r + (m_uf + 2*m_t)*(l_f + l_r))*9.8 - m_s*h*a)/(2*(l_f+l_r));

== matlab function Kalman_Project/MATLAB Function4 ==
  data: Fz output; a input; l_r data_store_memory; h data_store_memory; m_s data_store_memory; m_ur data_store_memory; l_f data_store_memory; m_t data_store_memory
function Fz = fcn(a)
global m_s m_ur l_f l_r h m_t;

Fz = ((m_s*l_f + (m_ur + 2*m_t)*(l_f + l_r))*9.8 + m_s*h*a)/(2*(l_f+l_r));

== matlab function Kalman_Project/MATLAB Function5 ==
  data: v_x input; w input; slip output; F_x input; F_z input; Reff data_store_memory; mu output
function [slip,mu] = fcn(v_x,w,F_x,F_z)
global Reff;

slip = (w*Reff - v_x)/max(v_x,w*Reff);
mu = F_x/F_z;

end
